simulink model "WSCC_Indian_400kV"  (R2022a)
settings: Solver=FixedStepDiscrete  StartTime=0.0  StopTime=1  FixedStep=5e-7  RelTol=1e-3
PreLoadFcn:
  | tf=1e-3
  | to=20e-3
model workspace (MAT data in the model file):
  tf = 0.001
  to = 0.02
undefined symbols (not defined in the file or in its folder): D1, Delta
libraries: spsFourierLib x72, spsThreePhaseVIMeasurementLib x21, spsThreePhaseBreakerLib x12, spsDistributedParametersLineLib x12, spsLoadFlowBusLib x9, spsThreePhaseParallelRLCLoadLib x6, spsThreePhaseSeriesRLCLoadLib x3, spsThreePhaseSourceLib x3, spsThreePhaseTransformerTwoWindingsLib x3, spsThreePhaseFaultLib x1, spspowerguiLib x1
(part 2 of 2)

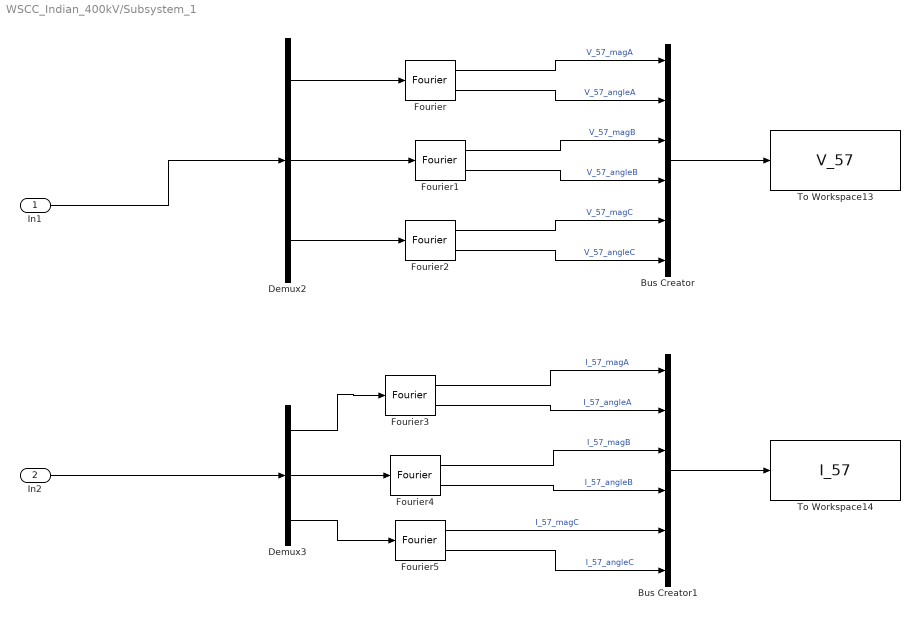
== system WSCC_Indian_400kV/Subsystem_1 ==
  In1 : Inport
  In2 : Inport  Port=2
  Bus Creator : BusCreator  Inputs=6
  Bus Creator1 : BusCreator  Inputs=6
  Demux2 : Demux  Outputs=3
  Demux3 : Demux  Outputs=3
  Fourier{,1..5} (6 alike) : spsFourierLib/Fourier  Freq=50  n=1  InInit=[0, 0]  Ts=tf
      settings: SourceProductBaseCode=PS
  To Workspace13 : ToWorkspace  VariableName=V_57  SaveFormat=Timeseries  SampleTime=to
  To Workspace14 : ToWorkspace  VariableName=I_57  SaveFormat=Timeseries  SampleTime=to
  wires:
  Demux3/3 -> Fourier5/1
  Demux3/2 -> Fourier4/1
  Demux3/1 -> Fourier3/1
  Demux2/2 -> Fourier1/1
  Demux2/3 -> Fourier2/1
  Demux2/1 -> Fourier/1
  In1/1 -> Demux2/1
  In2/1 -> Demux3/1
  Fourier/1 -> Bus Creator/1  "V_57_magA"
  Fourier/2 -> Bus Creator/2  "V_57_angleA"
  Fourier1/1 -> Bus Creator/3  "V_57_magB"
  Fourier1/2 -> Bus Creator/4  "V_57_angleB"
  Fourier2/1 -> Bus Creator/5  "V_57_magC"
  Fourier2/2 -> Bus Creator/6  "V_57_angleC"
  Bus Creator/1 -> To Workspace13/1
  Fourier3/1 -> Bus Creator1/1  "I_57_magA"
  Fourier3/2 -> Bus Creator1/2  "I_57_angleA"
  Fourier4/1 -> Bus Creator1/3  "I_57_magB"
  Fourier4/2 -> Bus Creator1/4  "I_57_angleB"
  Fourier5/1 -> Bus Creator1/5  "I_57_magC"
  Fourier5/2 -> Bus Creator1/6  "I_57_angleC"
  Bus Creator1/1 -> To Workspace14/1

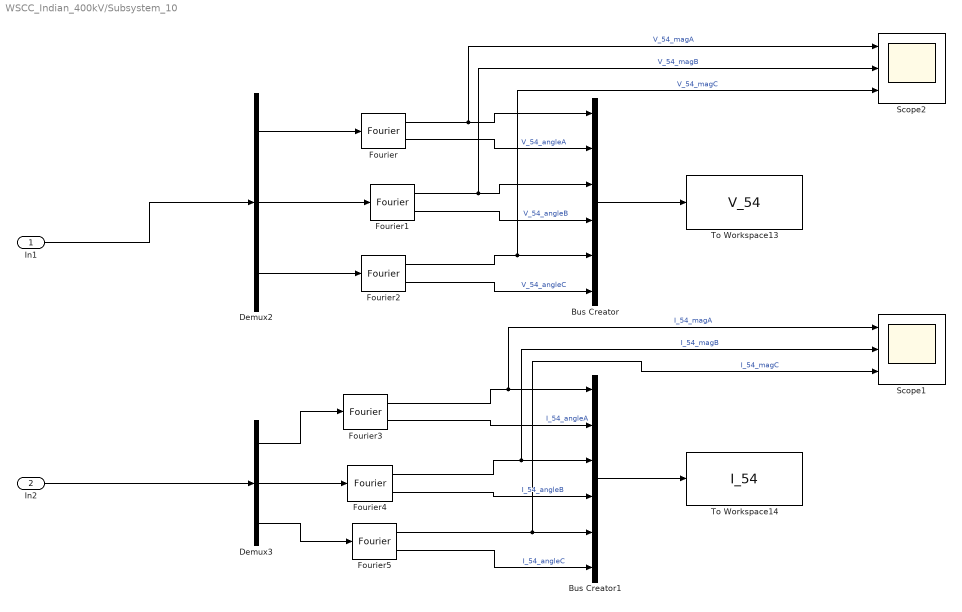
== system WSCC_Indian_400kV/Subsystem_10 ==
  In1 : Inport
  In2 : Inport  Port=2
  Bus Creator : BusCreator  Inputs=6
  Bus Creator1 : BusCreator  Inputs=6
  Demux2 : Demux  Outputs=3
  Demux3 : Demux  Outputs=3
  Fourier{,1..5} (6 alike) : spsFourierLib/Fourier  Freq=50  n=1  InInit=[0, 0]  Ts=tf
      settings: SourceProductBaseCode=PS
  Scope1 : Scope  NumInputPorts=3
  Scope2 : Scope  NumInputPorts=3
  To Workspace13 : ToWorkspace  VariableName=V_54  SaveFormat=Timeseries  SampleTime=to
  To Workspace14 : ToWorkspace  VariableName=I_54  SaveFormat=Timeseries  SampleTime=to
  wires:
  Demux3/3 -> Fourier5/1
  Demux3/2 -> Fourier4/1
  Demux3/1 -> Fourier3/1
  Demux2/2 -> Fourier1/1
  Demux2/3 -> Fourier2/1
  Demux2/1 -> Fourier/1
  In1/1 -> Demux2/1
  In2/1 -> Demux3/1
  Fourier/1 -> Scope2/1, Bus Creator/1  "V_54_magA"
  Fourier/2 -> Bus Creator/2  "V_54_angleA"
  Fourier1/1 -> Scope2/2, Bus Creator/3  "V_54_magB"
  Fourier1/2 -> Bus Creator/4  "V_54_angleB"
  Fourier2/1 -> Scope2/3, Bus Creator/5  "V_54_magC"
  Fourier2/2 -> Bus Creator/6  "V_54_angleC"
  Bus Creator/1 -> To Workspace13/1
  Fourier3/1 -> Scope1/1, Bus Creator1/1  "I_54_magA"
  Fourier3/2 -> Bus Creator1/2  "I_54_angleA"
  Fourier4/1 -> Scope1/2, Bus Creator1/3  "I_54_magB"
  Fourier4/2 -> Bus Creator1/4  "I_54_angleB"
  Fourier5/1 -> Scope1/3, Bus Creator1/5  "I_54_magC"
  Fourier5/2 -> Bus Creator1/6  "I_54_angleC"
  Bus Creator1/1 -> To Workspace14/1

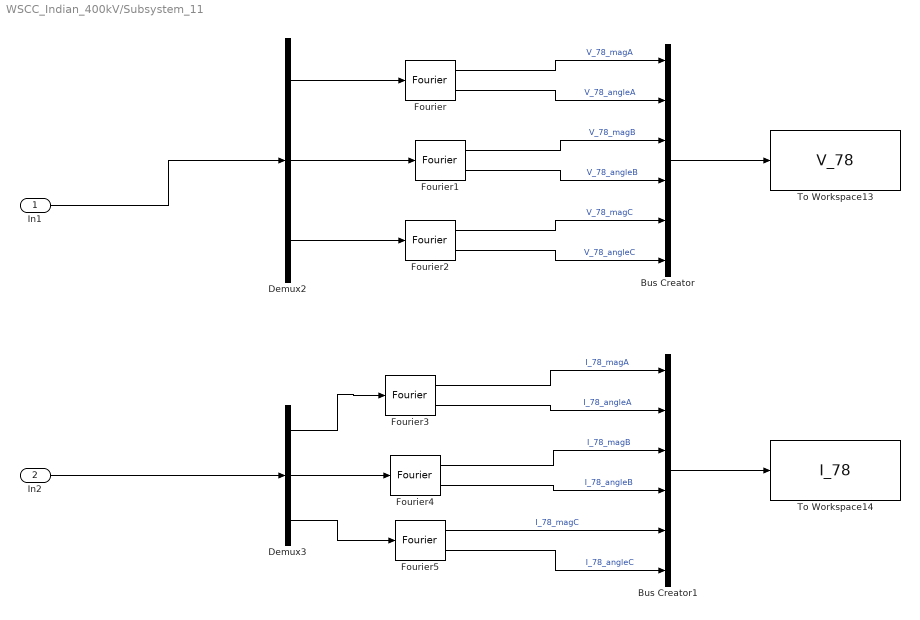
== system WSCC_Indian_400kV/Subsystem_11 ==
  In1 : Inport
  In2 : Inport  Port=2
  Bus Creator : BusCreator  Inputs=6
  Bus Creator1 : BusCreator  Inputs=6
  Demux2 : Demux  Outputs=3
  Demux3 : Demux  Outputs=3
  Fourier{,1..5} (6 alike) : spsFourierLib/Fourier  Freq=50  n=1  InInit=[0, 0]  Ts=tf
      settings: SourceProductBaseCode=PS
  To Workspace13 : ToWorkspace  VariableName=V_78  SaveFormat=Timeseries  SampleTime=to
  To Workspace14 : ToWorkspace  VariableName=I_78  SaveFormat=Timeseries  SampleTime=to
  wires:
  Demux3/3 -> Fourier5/1
  Demux3/2 -> Fourier4/1
  Demux3/1 -> Fourier3/1
  Demux2/2 -> Fourier1/1
  Demux2/3 -> Fourier2/1
  Demux2/1 -> Fourier/1
  In1/1 -> Demux2/1
  In2/1 -> Demux3/1
  Fourier/1 -> Bus Creator/1  "V_78_magA"
  Fourier/2 -> Bus Creator/2  "V_78_angleA"
  Fourier1/1 -> Bus Creator/3  "V_78_magB"
  Fourier1/2 -> Bus Creator/4  "V_78_angleB"
  Fourier2/1 -> Bus Creator/5  "V_78_magC"
  Fourier2/2 -> Bus Creator/6  "V_78_angleC"
  Bus Creator/1 -> To Workspace13/1
  Fourier3/1 -> Bus Creator1/1  "I_78_magA"
  Fourier3/2 -> Bus Creator1/2  "I_78_angleA"
  Fourier4/1 -> Bus Creator1/3  "I_78_magB"
  Fourier4/2 -> Bus Creator1/4  "I_78_angleB"
  Fourier5/1 -> Bus Creator1/5  "I_78_magC"
  Fourier5/2 -> Bus Creator1/6  "I_78_angleC"
  Bus Creator1/1 -> To Workspace14/1

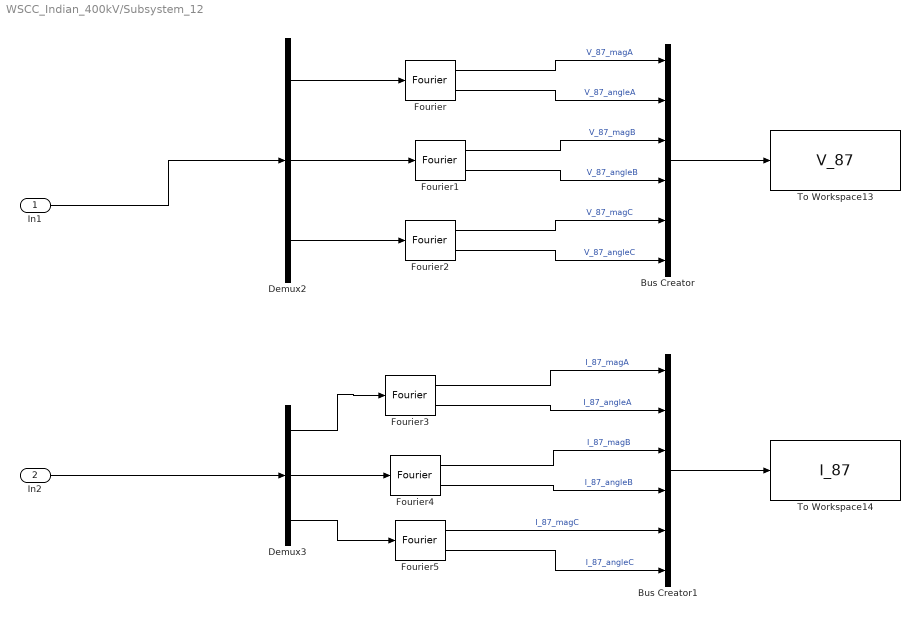
== system WSCC_Indian_400kV/Subsystem_12 ==
  In1 : Inport
  In2 : Inport  Port=2
  Bus Creator : BusCreator  Inputs=6
  Bus Creator1 : BusCreator  Inputs=6
  Demux2 : Demux  Outputs=3
  Demux3 : Demux  Outputs=3
  Fourier{,1..5} (6 alike) : spsFourierLib/Fourier  Freq=50  n=1  InInit=[0, 0]  Ts=tf
      settings: SourceProductBaseCode=PS
  To Workspace13 : ToWorkspace  VariableName=V_87  SaveFormat=Timeseries  SampleTime=to
  To Workspace14 : ToWorkspace  VariableName=I_87  SaveFormat=Timeseries  SampleTime=to
  wires:
  Demux3/3 -> Fourier5/1
  Demux3/2 -> Fourier4/1
  Demux3/1 -> Fourier3/1
  Demux2/2 -> Fourier1/1
  Demux2/3 -> Fourier2/1
  Demux2/1 -> Fourier/1
  In1/1 -> Demux2/1
  In2/1 -> Demux3/1
  Fourier/1 -> Bus Creator/1  "V_87_magA"
  Fourier/2 -> Bus Creator/2  "V_87_angleA"
  Fourier1/1 -> Bus Creator/3  "V_87_magB"
  Fourier1/2 -> Bus Creator/4  "V_87_angleB"
  Fourier2/1 -> Bus Creator/5  "V_87_magC"
  Fourier2/2 -> Bus Creator/6  "V_87_angleC"
  Bus Creator/1 -> To Workspace13/1
  Fourier3/1 -> Bus Creator1/1  "I_87_magA"
  Fourier3/2 -> Bus Creator1/2  "I_87_angleA"
  Fourier4/1 -> Bus Creator1/3  "I_87_magB"
  Fourier4/2 -> Bus Creator1/4  "I_87_angleB"
  Fourier5/1 -> Bus Creator1/5  "I_87_magC"
  Fourier5/2 -> Bus Creator1/6  "I_87_angleC"
  Bus Creator1/1 -> To Workspace14/1

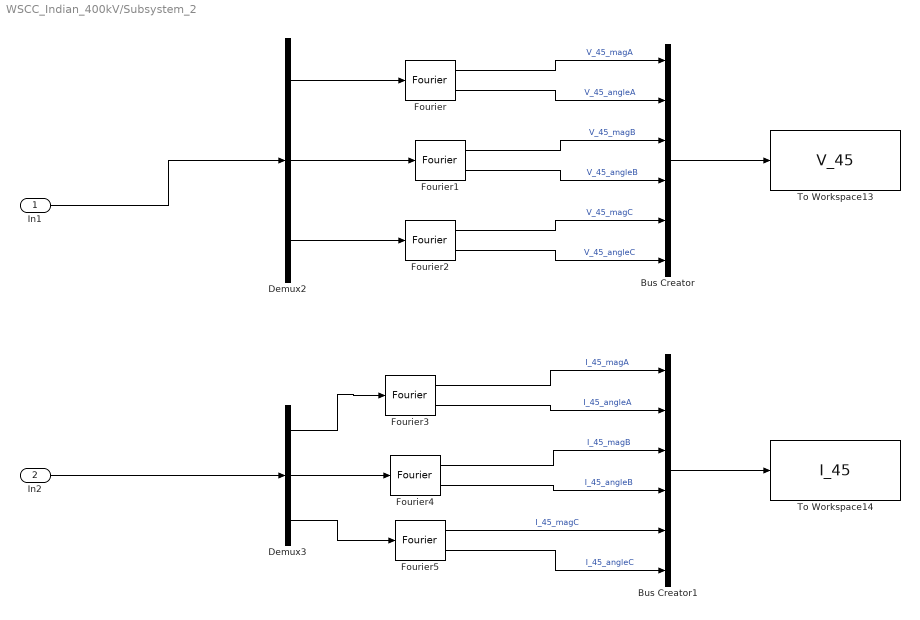
== system WSCC_Indian_400kV/Subsystem_2 ==
  In1 : Inport
  In2 : Inport  Port=2
  Bus Creator : BusCreator  Inputs=6
  Bus Creator1 : BusCreator  Inputs=6
  Demux2 : Demux  Outputs=3
  Demux3 : Demux  Outputs=3
  Fourier{,1..5} (6 alike) : spsFourierLib/Fourier  Freq=50  n=1  InInit=[0, 0]  Ts=tf
      settings: SourceProductBaseCode=PS
  To Workspace13 : ToWorkspace  VariableName=V_45  SaveFormat=Timeseries  SampleTime=to
  To Workspace14 : ToWorkspace  VariableName=I_45  SaveFormat=Timeseries  SampleTime=to
  wires:
  Demux3/3 -> Fourier5/1
  Demux3/2 -> Fourier4/1
  Demux3/1 -> Fourier3/1
  Demux2/2 -> Fourier1/1
  Demux2/3 -> Fourier2/1
  Demux2/1 -> Fourier/1
  In1/1 -> Demux2/1
  In2/1 -> Demux3/1
  Fourier/1 -> Bus Creator/1  "V_45_magA"
  Fourier/2 -> Bus Creator/2  "V_45_angleA"
  Fourier1/1 -> Bus Creator/3  "V_45_magB"
  Fourier1/2 -> Bus Creator/4  "V_45_angleB"
  Fourier2/1 -> Bus Creator/5  "V_45_magC"
  Fourier2/2 -> Bus Creator/6  "V_45_angleC"
  Bus Creator/1 -> To Workspace13/1
  Fourier3/1 -> Bus Creator1/1  "I_45_magA"
  Fourier3/2 -> Bus Creator1/2  "I_45_angleA"
  Fourier4/1 -> Bus Creator1/3  "I_45_magB"
  Fourier4/2 -> Bus Creator1/4  "I_45_angleB"
  Fourier5/1 -> Bus Creator1/5  "I_45_magC"
  Fourier5/2 -> Bus Creator1/6  "I_45_angleC"
  Bus Creator1/1 -> To Workspace14/1

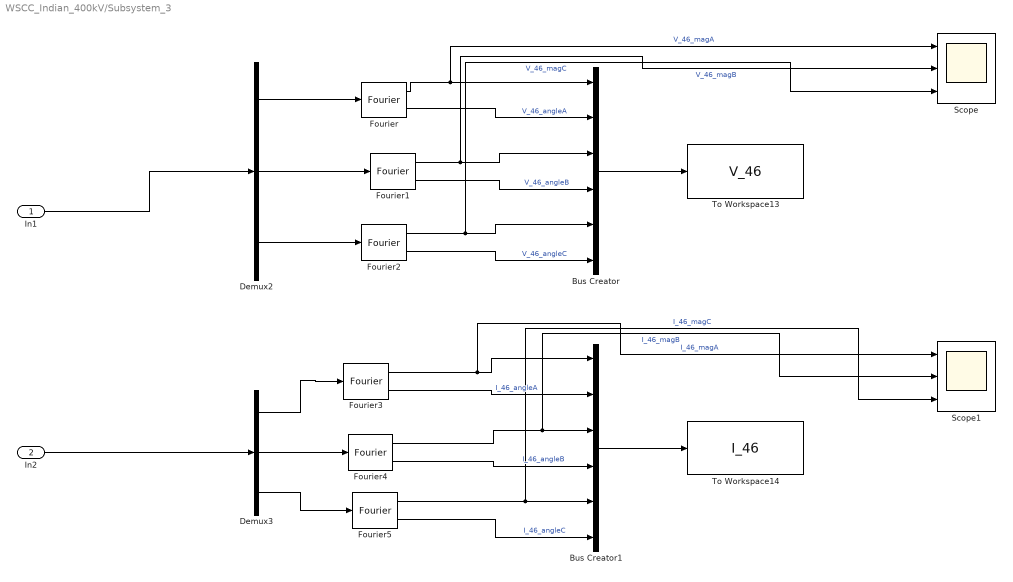
== system WSCC_Indian_400kV/Subsystem_3 ==
  In1 : Inport
  In2 : Inport  Port=2
  Bus Creator : BusCreator  Inputs=6
  Bus Creator1 : BusCreator  Inputs=6
  Demux2 : Demux  Outputs=3
  Demux3 : Demux  Outputs=3
  Fourier{,1..5} (6 alike) : spsFourierLib/Fourier  Freq=50  n=1  InInit=[0, 0]  Ts=tf
      settings: SourceProductBaseCode=PS
  Scope : Scope  NumInputPorts=3
  Scope1 : Scope  NumInputPorts=3
  To Workspace13 : ToWorkspace  VariableName=V_46  SaveFormat=Timeseries  SampleTime=to
  To Workspace14 : ToWorkspace  VariableName=I_46  SaveFormat=Timeseries  SampleTime=to
  wires:
  Demux3/3 -> Fourier5/1
  Demux3/2 -> Fourier4/1
  Demux3/1 -> Fourier3/1
  Demux2/2 -> Fourier1/1
  Demux2/3 -> Fourier2/1
  Demux2/1 -> Fourier/1
  In1/1 -> Demux2/1
  In2/1 -> Demux3/1
  Fourier/1 -> Scope/1, Bus Creator/1  "V_46_magA"
  Fourier/2 -> Bus Creator/2  "V_46_angleA"
  Fourier1/1 -> Scope/2, Bus Creator/3  "V_46_magB"
  Fourier1/2 -> Bus Creator/4  "V_46_angleB"
  Fourier2/1 -> Scope/3, Bus Creator/5  "V_46_magC"
  Fourier2/2 -> Bus Creator/6  "V_46_angleC"
  Bus Creator/1 -> To Workspace13/1
  Fourier3/1 -> Scope1/1, Bus Creator1/1  "I_46_magA"
  Fourier3/2 -> Bus Creator1/2  "I_46_angleA"
  Fourier4/1 -> Scope1/2, Bus Creator1/3  "I_46_magB"
  Fourier4/2 -> Bus Creator1/4  "I_46_angleB"
  Fourier5/1 -> Scope1/3, Bus Creator1/5  "I_46_magC"
  Fourier5/2 -> Bus Creator1/6  "I_46_angleC"
  Bus Creator1/1 -> To Workspace14/1

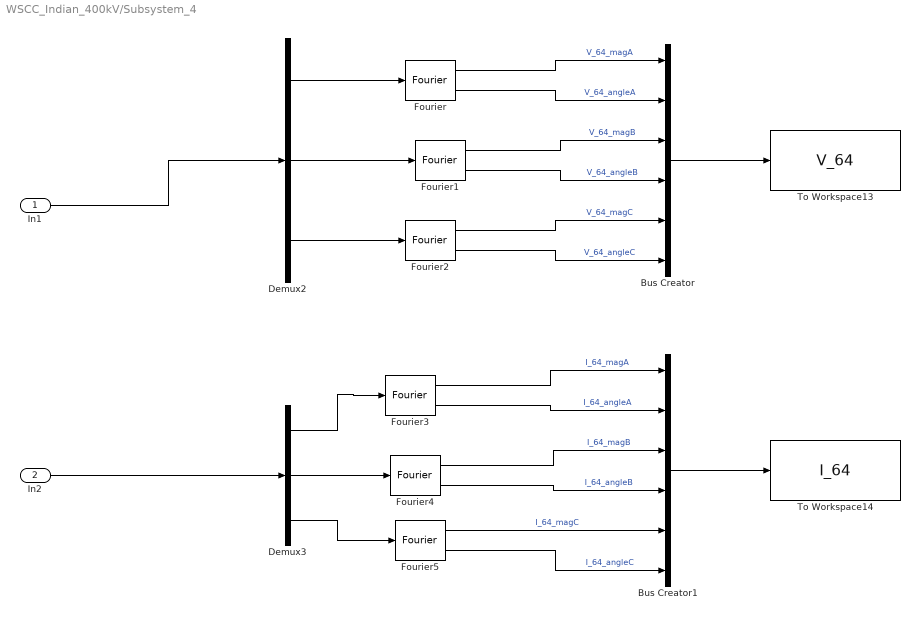
== system WSCC_Indian_400kV/Subsystem_4 ==
  In1 : Inport
  In2 : Inport  Port=2
  Bus Creator : BusCreator  Inputs=6
  Bus Creator1 : BusCreator  Inputs=6
  Demux2 : Demux  Outputs=3
  Demux3 : Demux  Outputs=3
  Fourier{,1..5} (6 alike) : spsFourierLib/Fourier  Freq=50  n=1  InInit=[0, 0]  Ts=tf
      settings: SourceProductBaseCode=PS
  To Workspace13 : ToWorkspace  VariableName=V_64  SaveFormat=Timeseries  SampleTime=to
  To Workspace14 : ToWorkspace  VariableName=I_64  SaveFormat=Timeseries  SampleTime=to
  wires:
  Demux3/3 -> Fourier5/1
  Demux3/2 -> Fourier4/1
  Demux3/1 -> Fourier3/1
  Demux2/2 -> Fourier1/1
  Demux2/3 -> Fourier2/1
  Demux2/1 -> Fourier/1
  In1/1 -> Demux2/1
  In2/1 -> Demux3/1
  Fourier/1 -> Bus Creator/1  "V_64_magA"
  Fourier/2 -> Bus Creator/2  "V_64_angleA"
  Fourier1/1 -> Bus Creator/3  "V_64_magB"
  Fourier1/2 -> Bus Creator/4  "V_64_angleB"
  Fourier2/1 -> Bus Creator/5  "V_64_magC"
  Fourier2/2 -> Bus Creator/6  "V_64_angleC"
  Bus Creator/1 -> To Workspace13/1
  Fourier3/1 -> Bus Creator1/1  "I_64_magA"
  Fourier3/2 -> Bus Creator1/2  "I_64_angleA"
  Fourier4/1 -> Bus Creator1/3  "I_64_magB"
  Fourier4/2 -> Bus Creator1/4  "I_64_angleB"
  Fourier5/1 -> Bus Creator1/5  "I_64_magC"
  Fourier5/2 -> Bus Creator1/6  "I_64_angleC"
  Bus Creator1/1 -> To Workspace14/1

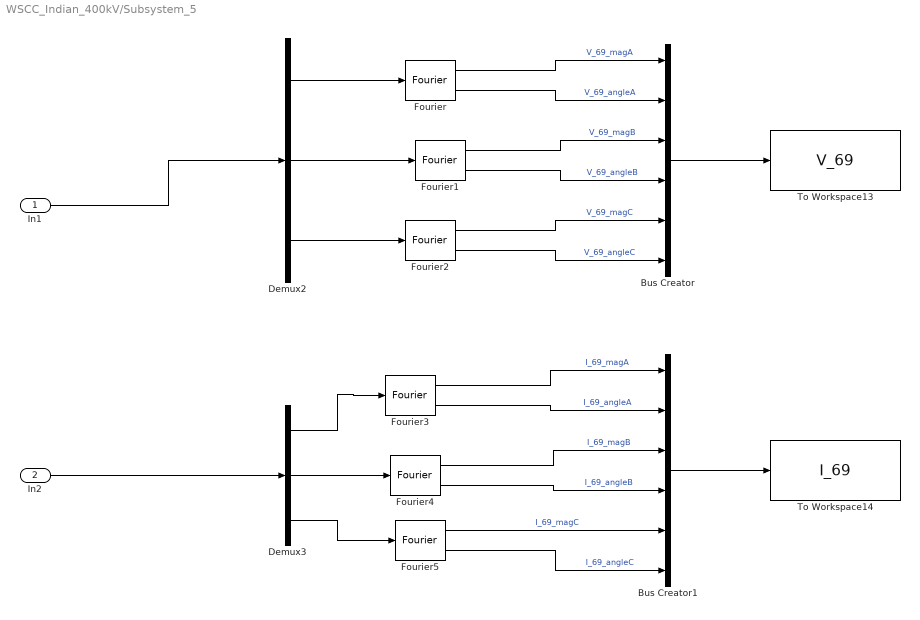
== system WSCC_Indian_400kV/Subsystem_5 ==
  In1 : Inport
  In2 : Inport  Port=2
  Bus Creator : BusCreator  Inputs=6
  Bus Creator1 : BusCreator  Inputs=6
  Demux2 : Demux  Outputs=3
  Demux3 : Demux  Outputs=3
  Fourier{,1..5} (6 alike) : spsFourierLib/Fourier  Freq=50  n=1  InInit=[0, 0]  Ts=tf
      settings: SourceProductBaseCode=PS
  To Workspace13 : ToWorkspace  VariableName=V_69  SaveFormat=Timeseries  SampleTime=to
  To Workspace14 : ToWorkspace  VariableName=I_69  SaveFormat=Timeseries  SampleTime=to
  wires:
  Demux3/3 -> Fourier5/1
  Demux3/2 -> Fourier4/1
  Demux3/1 -> Fourier3/1
  Demux2/2 -> Fourier1/1
  Demux2/3 -> Fourier2/1
  Demux2/1 -> Fourier/1
  In1/1 -> Demux2/1
  In2/1 -> Demux3/1
  Fourier/1 -> Bus Creator/1  "V_69_magA"
  Fourier/2 -> Bus Creator/2  "V_69_angleA"
  Fourier1/1 -> Bus Creator/3  "V_69_magB"
  Fourier1/2 -> Bus Creator/4  "V_69_angleB"
  Fourier2/1 -> Bus Creator/5  "V_69_magC"
  Fourier2/2 -> Bus Creator/6  "V_69_angleC"
  Bus Creator/1 -> To Workspace13/1
  Fourier3/1 -> Bus Creator1/1  "I_69_magA"
  Fourier3/2 -> Bus Creator1/2  "I_69_angleA"
  Fourier4/1 -> Bus Creator1/3  "I_69_magB"
  Fourier4/2 -> Bus Creator1/4  "I_69_angleB"
  Fourier5/1 -> Bus Creator1/5  "I_69_magC"
  Fourier5/2 -> Bus Creator1/6  "I_69_angleC"
  Bus Creator1/1 -> To Workspace14/1

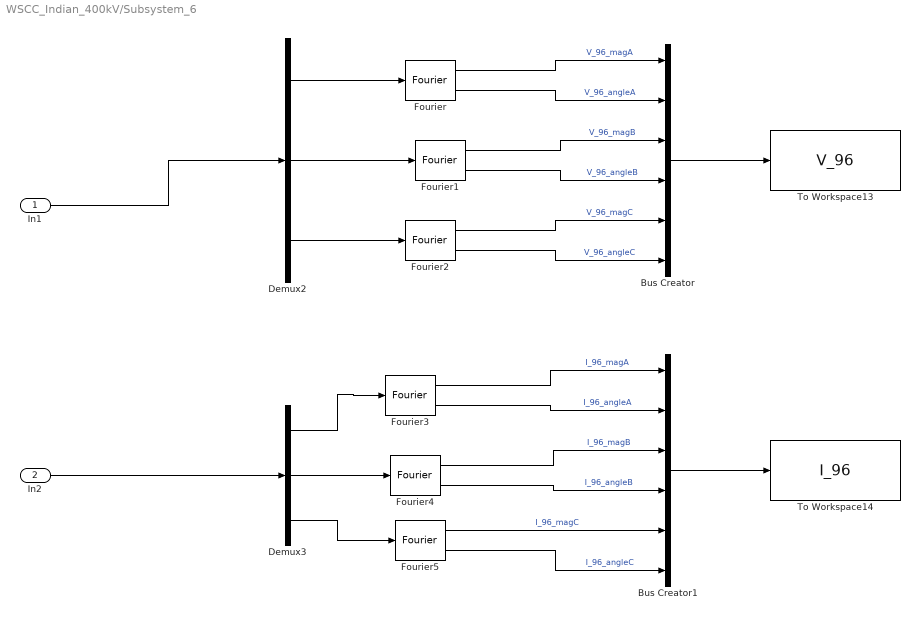
== system WSCC_Indian_400kV/Subsystem_6 ==
  In1 : Inport
  In2 : Inport  Port=2
  Bus Creator : BusCreator  Inputs=6
  Bus Creator1 : BusCreator  Inputs=6
  Demux2 : Demux  Outputs=3
  Demux3 : Demux  Outputs=3
  Fourier{,1..5} (6 alike) : spsFourierLib/Fourier  Freq=50  n=1  InInit=[0, 0]  Ts=tf
      settings: SourceProductBaseCode=PS
  To Workspace13 : ToWorkspace  VariableName=V_96  SaveFormat=Timeseries  SampleTime=to
  To Workspace14 : ToWorkspace  VariableName=I_96  SaveFormat=Timeseries  SampleTime=to
  wires:
  Demux3/3 -> Fourier5/1
  Demux3/2 -> Fourier4/1
  Demux3/1 -> Fourier3/1
  Demux2/2 -> Fourier1/1
  Demux2/3 -> Fourier2/1
  Demux2/1 -> Fourier/1
  In1/1 -> Demux2/1
  In2/1 -> Demux3/1
  Fourier/1 -> Bus Creator/1  "V_96_magA"
  Fourier/2 -> Bus Creator/2  "V_96_angleA"
  Fourier1/1 -> Bus Creator/3  "V_96_magB"
  Fourier1/2 -> Bus Creator/4  "V_96_angleB"
  Fourier2/1 -> Bus Creator/5  "V_96_magC"
  Fourier2/2 -> Bus Creator/6  "V_96_angleC"
  Bus Creator/1 -> To Workspace13/1
  Fourier3/1 -> Bus Creator1/1  "I_96_magA"
  Fourier3/2 -> Bus Creator1/2  "I_96_angleA"
  Fourier4/1 -> Bus Creator1/3  "I_96_magB"
  Fourier4/2 -> Bus Creator1/4  "I_96_angleB"
  Fourier5/1 -> Bus Creator1/5  "I_96_magC"
  Fourier5/2 -> Bus Creator1/6  "I_96_angleC"
  Bus Creator1/1 -> To Workspace14/1

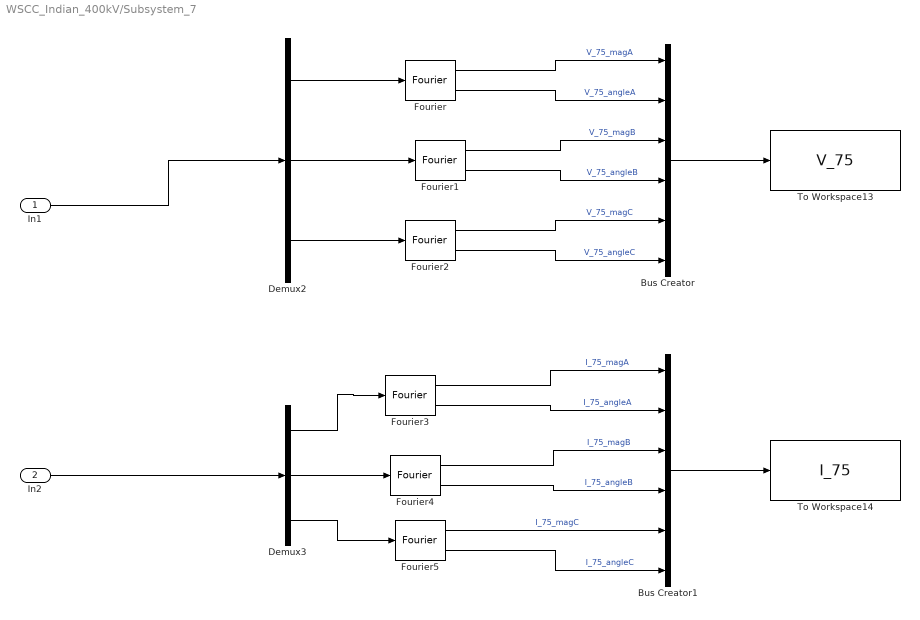
== system WSCC_Indian_400kV/Subsystem_7 ==
  In1 : Inport
  In2 : Inport  Port=2
  Bus Creator : BusCreator  Inputs=6
  Bus Creator1 : BusCreator  Inputs=6
  Demux2 : Demux  Outputs=3
  Demux3 : Demux  Outputs=3
  Fourier{,1..5} (6 alike) : spsFourierLib/Fourier  Freq=50  n=1  InInit=[0, 0]  Ts=tf
      settings: SourceProductBaseCode=PS
  To Workspace13 : ToWorkspace  VariableName=V_75  SaveFormat=Timeseries  SampleTime=to
  To Workspace14 : ToWorkspace  VariableName=I_75  SaveFormat=Timeseries  SampleTime=to
  wires:
  Demux3/3 -> Fourier5/1
  Demux3/2 -> Fourier4/1
  Demux3/1 -> Fourier3/1
  Demux2/2 -> Fourier1/1
  Demux2/3 -> Fourier2/1
  Demux2/1 -> Fourier/1
  In1/1 -> Demux2/1
  In2/1 -> Demux3/1
  Fourier/1 -> Bus Creator/1  "V_75_magA"
  Fourier/2 -> Bus Creator/2  "V_75_angleA"
  Fourier1/1 -> Bus Creator/3  "V_75_magB"
  Fourier1/2 -> Bus Creator/4  "V_75_angleB"
  Fourier2/1 -> Bus Creator/5  "V_75_magC"
  Fourier2/2 -> Bus Creator/6  "V_75_angleC"
  Bus Creator/1 -> To Workspace13/1
  Fourier3/1 -> Bus Creator1/1  "I_75_magA"
  Fourier3/2 -> Bus Creator1/2  "I_75_angleA"
  Fourier4/1 -> Bus Creator1/3  "I_75_magB"
  Fourier4/2 -> Bus Creator1/4  "I_75_angleB"
  Fourier5/1 -> Bus Creator1/5  "I_75_magC"
  Fourier5/2 -> Bus Creator1/6  "I_75_angleC"
  Bus Creator1/1 -> To Workspace14/1

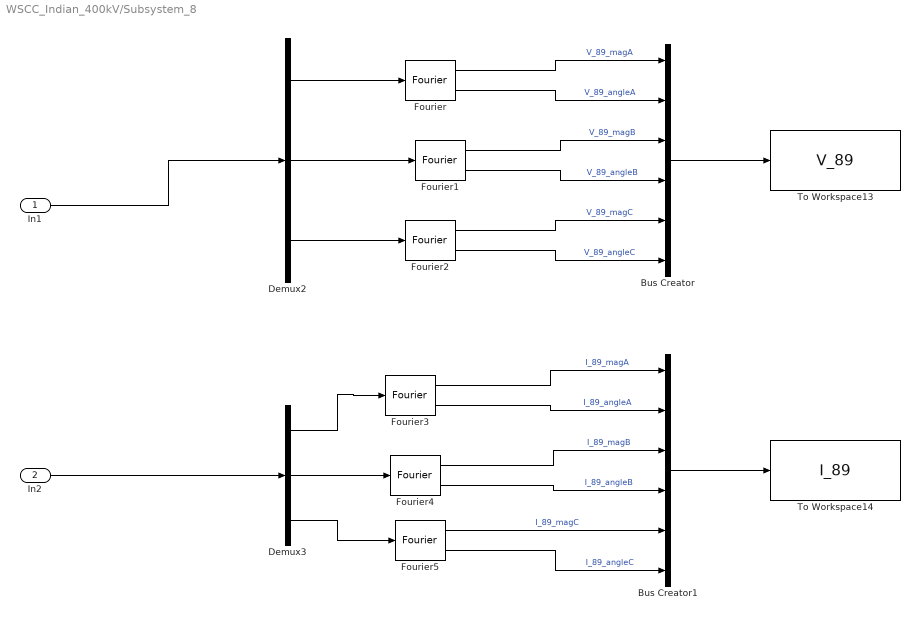
== system WSCC_Indian_400kV/Subsystem_8 ==
  In1 : Inport
  In2 : Inport  Port=2
  Bus Creator : BusCreator  Inputs=6
  Bus Creator1 : BusCreator  Inputs=6
  Demux2 : Demux  Outputs=3
  Demux3 : Demux  Outputs=3
  Fourier{,1..5} (6 alike) : spsFourierLib/Fourier  Freq=50  n=1  InInit=[0, 0]  Ts=tf
      settings: SourceProductBaseCode=PS
  To Workspace13 : ToWorkspace  VariableName=V_89  SaveFormat=Timeseries  SampleTime=to
  To Workspace14 : ToWorkspace  VariableName=I_89  SaveFormat=Timeseries  SampleTime=to
  wires:
  Demux3/3 -> Fourier5/1
  Demux3/2 -> Fourier4/1
  Demux3/1 -> Fourier3/1
  Demux2/2 -> Fourier1/1
  Demux2/3 -> Fourier2/1
  Demux2/1 -> Fourier/1
  In1/1 -> Demux2/1
  In2/1 -> Demux3/1
  Fourier/1 -> Bus Creator/1  "V_89_magA"
  Fourier/2 -> Bus Creator/2  "V_89_angleA"
  Fourier1/1 -> Bus Creator/3  "V_89_magB"
  Fourier1/2 -> Bus Creator/4  "V_89_angleB"
  Fourier2/1 -> Bus Creator/5  "V_89_magC"
  Fourier2/2 -> Bus Creator/6  "V_89_angleC"
  Bus Creator/1 -> To Workspace13/1
  Fourier3/1 -> Bus Creator1/1  "I_89_magA"
  Fourier3/2 -> Bus Creator1/2  "I_89_angleA"
  Fourier4/1 -> Bus Creator1/3  "I_89_magB"
  Fourier4/2 -> Bus Creator1/4  "I_89_angleB"
  Fourier5/1 -> Bus Creator1/5  "I_89_magC"
  Fourier5/2 -> Bus Creator1/6  "I_89_angleC"
  Bus Creator1/1 -> To Workspace14/1

== system WSCC_Indian_400kV/Subsystem_9 ==
  In1 : Inport
  In2 : Inport  Port=2
  Bus Creator : BusCreator  Inputs=6
  Bus Creator1 : BusCreator  Inputs=6
  Demux2 : Demux  Outputs=3
  Demux3 : Demux  Outputs=3
  Fourier{,1..5} (6 alike) : spsFourierLib/Fourier  Freq=50  n=1  InInit=[0, 0]  Ts=tf
      settings: SourceProductBaseCode=PS
  To Workspace13 : ToWorkspace  VariableName=V_98  SaveFormat=Timeseries  SampleTime=to
  To Workspace14 : ToWorkspace  VariableName=I_98  SaveFormat=Timeseries  SampleTime=to
  wires:
  Demux3/3 -> Fourier5/1
  Demux3/2 -> Fourier4/1
  Demux3/1 -> Fourier3/1
  Demux2/2 -> Fourier1/1
  Demux2/3 -> Fourier2/1
  Demux2/1 -> Fourier/1
  In1/1 -> Demux2/1
  In2/1 -> Demux3/1
  Fourier/1 -> Bus Creator/1  "V_98_magA"
  Fourier/2 -> Bus Creator/2  "V_98_angleA"
  Fourier1/1 -> Bus Creator/3  "V_98_magB"
  Fourier1/2 -> Bus Creator/4  "V_98_angleB"
  Fourier2/1 -> Bus Creator/5  "V_98_magC"
  Fourier2/2 -> Bus Creator/6  "V_98_angleC"
  Bus Creator/1 -> To Workspace13/1
  Fourier3/1 -> Bus Creator1/1  "I_98_magA"
  Fourier3/2 -> Bus Creator1/2  "I_98_angleA"
  Fourier4/1 -> Bus Creator1/3  "I_98_magB"
  Fourier4/2 -> Bus Creator1/4  "I_98_angleB"
  Fourier5/1 -> Bus Creator1/5  "I_98_magC"
  Fourier5/2 -> Bus Creator1/6  "I_98_angleC"
  Bus Creator1/1 -> To Workspace14/1
